simulink model "meart_trace60"  (Simulink 6.5)
settings: Solver=FixedStepDiscrete  StartTime=0.0  StopTime=5  FixedStep=0.0005  RelTol=1e-3
undefined symbols (not defined in the file or in its folder): MF, PD2
libraries: xpcueilib x1
settings Model: Creator=cdfz  LastModifiedBy=avnerw  TunableVars=threshold  TunableVarsStorageClass=Auto  BufferReuse=off  ProdHWDeviceType=32-bit xPC Target (AMD Athlon)
settings ConfigSet: SimulationMode=external
settings DataIOCC: LimitDataPoints=off  SignalLogging=off  SaveTime=off
settings OptimizationCC: BlockReduction=off  InlineParams=on  OptimizeBlockIOStorage=off  BufferReuse=off  EnforceIntegerDowncast=off  ExpressionFolding=off  LocalBlockOutputs=off  EfficientFloat2IntCast=on
settings HardwareCC: ProdIntDivRoundTo=Zero  ProdEndianess=LittleEndian  ProdHWDeviceType=32-bit xPC Target (AMD Athlon)
settings RTWCC: SystemTargetFile=xpctarget.tlc  TemplateMakefile=xpc_default_tmf  Description=xPC Target  ProcessScript=xpctarget_make_rtw_hook
settings xpcTargetCC: TargetFcnLib=ansi_tfl_tmw.mat  GenFloatMathFcnCalls=ANSI_C  ExtModeInterfaceLevel=Level2 - Open  RL32LogBufSizeModifier=3*2000*3600  RL32IRQSourceModifier=10  xPCIRQSourceBoard=UEI_MFx

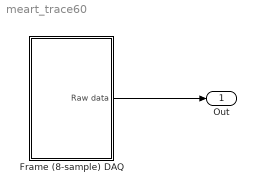
== system meart_trace60 ==
  Frame (8-sample) DAQ : Subsystem  TreatAsAtomicUnit=on  mask{frametime=0.0005}
  Out : Outport
  wires:
  Frame (8-sample) DAQ/1(Raw data) -> Out/1

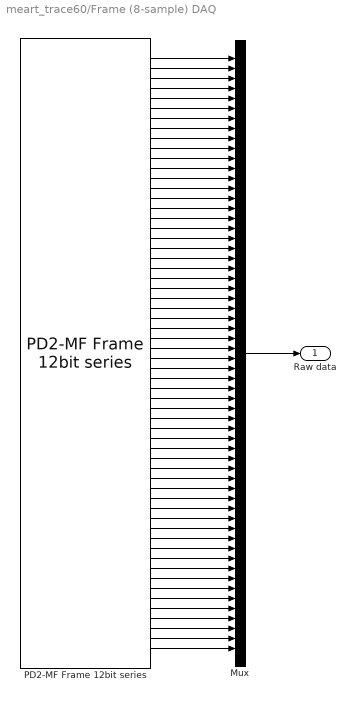
== system meart_trace60/Frame (8-sample) DAQ ==
  Mux : Mux  Inputs=60
  "PD2-MF Frame 12bit series " : xpcueilib/A//D Frame/PD2-MF Frame 12bit series   boardtypein=PD2-MF-64-3M/12H  channel=[1:60]  gain=[1]  mux=[1]  range=+- 5 Volts  sediff=Single Ended  framesize=8  outfmt=Vector  clsource=Internal  scantime=-1  frametime=frametime  sampletime=off  slave=off  freq=8/frametime*60  burst=32  pcislot=-1
  Raw data : Outport
  wires:
  Mux/1 -> Raw data/1
  "PD2-MF Frame 12bit series "/60 -> Mux/60
  "PD2-MF Frame 12bit series "/59 -> Mux/59
  "PD2-MF Frame 12bit series "/58 -> Mux/58
  "PD2-MF Frame 12bit series "/57 -> Mux/57
  "PD2-MF Frame 12bit series "/56 -> Mux/56
  "PD2-MF Frame 12bit series "/55 -> Mux/55
  "PD2-MF Frame 12bit series "/54 -> Mux/54
  "PD2-MF Frame 12bit series "/53 -> Mux/53
  "PD2-MF Frame 12bit series "/52 -> Mux/52
  "PD2-MF Frame 12bit series "/51 -> Mux/51
  "PD2-MF Frame 12bit series "/50 -> Mux/50
  "PD2-MF Frame 12bit series "/49 -> Mux/49
  "PD2-MF Frame 12bit series "/48 -> Mux/48
  "PD2-MF Frame 12bit series "/47 -> Mux/47
  "PD2-MF Frame 12bit series "/46 -> Mux/46
  "PD2-MF Frame 12bit series "/45 -> Mux/45
  "PD2-MF Frame 12bit series "/44 -> Mux/44
  "PD2-MF Frame 12bit series "/43 -> Mux/43
  "PD2-MF Frame 12bit series "/42 -> Mux/42
  "PD2-MF Frame 12bit series "/41 -> Mux/41
  "PD2-MF Frame 12bit series "/40 -> Mux/40
  "PD2-MF Frame 12bit series "/39 -> Mux/39
  "PD2-MF Frame 12bit series "/38 -> Mux/38
  "PD2-MF Frame 12bit series "/37 -> Mux/37
  "PD2-MF Frame 12bit series "/36 -> Mux/36
  "PD2-MF Frame 12bit series "/35 -> Mux/35
  "PD2-MF Frame 12bit series "/34 -> Mux/34
  "PD2-MF Frame 12bit series "/33 -> Mux/33
  "PD2-MF Frame 12bit series "/32 -> Mux/32
  "PD2-MF Frame 12bit series "/31 -> Mux/31
  "PD2-MF Frame 12bit series "/30 -> Mux/30
  "PD2-MF Frame 12bit series "/29 -> Mux/29
  "PD2-MF Frame 12bit series "/28 -> Mux/28
  "PD2-MF Frame 12bit series "/27 -> Mux/27
  "PD2-MF Frame 12bit series "/26 -> Mux/26
  "PD2-MF Frame 12bit series "/25 -> Mux/25
  "PD2-MF Frame 12bit series "/24 -> Mux/24
  "PD2-MF Frame 12bit series "/23 -> Mux/23
  "PD2-MF Frame 12bit series "/22 -> Mux/22
  "PD2-MF Frame 12bit series "/21 -> Mux/21
  "PD2-MF Frame 12bit series "/20 -> Mux/20
  "PD2-MF Frame 12bit series "/19 -> Mux/19
  "PD2-MF Frame 12bit series "/18 -> Mux/18
  "PD2-MF Frame 12bit series "/17 -> Mux/17
  "PD2-MF Frame 12bit series "/16 -> Mux/16
  "PD2-MF Frame 12bit series "/15 -> Mux/15
  "PD2-MF Frame 12bit series "/14 -> Mux/14
  "PD2-MF Frame 12bit series "/13 -> Mux/13
  "PD2-MF Frame 12bit series "/12 -> Mux/12
  "PD2-MF Frame 12bit series "/11 -> Mux/11
  "PD2-MF Frame 12bit series "/10 -> Mux/10
  "PD2-MF Frame 12bit series "/9 -> Mux/9
  "PD2-MF Frame 12bit series "/8 -> Mux/8
  "PD2-MF Frame 12bit series "/7 -> Mux/7
  "PD2-MF Frame 12bit series "/6 -> Mux/6
  "PD2-MF Frame 12bit series "/5 -> Mux/5
  "PD2-MF Frame 12bit series "/3 -> Mux/3
  "PD2-MF Frame 12bit series "/4 -> Mux/4
  "PD2-MF Frame 12bit series "/2 -> Mux/2
  "PD2-MF Frame 12bit series "/1 -> Mux/1
